simulink model "simulation"  (R2016a)
settings: Solver=VariableStepAuto  StartTime=0.0  StopTime=0.4  MaxStep=0.01  RelTol=1e-4
settings Model: Creator=michael  LastModifiedBy=michael
settings DataIOCC: LimitDataPoints=on  SaveOutput=off  SaveTime=off
settings OptimizationCC: ExpressionDepthLimit=2147483647  LifeSpan=1
settings DebuggingCC: UnderspecifiedInitializationDetection=Classic  MergeDetectMultiDrivingBlocksExec=none  FcnCallInpInsideContextMsg=EnableAllAsWarning  AllowSymbolicDim=off  StateNameClashWarn=warning
settings GRTTargetCC: CombineOutputUpdateFcns=off  GRTInterface=on

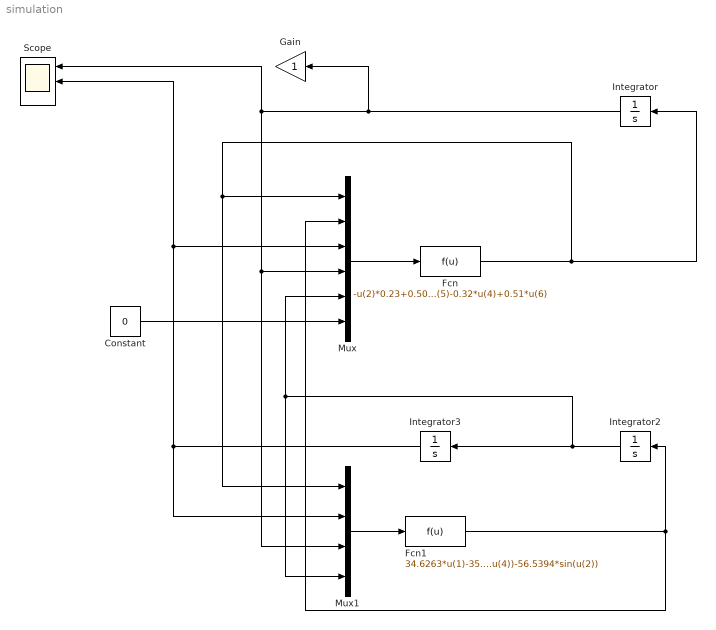
== system simulation ==
  Constant : Constant  Value=0
  Fcn : Fcn  Expr=-u(2)*0.23+0.505*(2*cos(u(3))-u(5)*sin(2*u(3))/cos(u(3)))+0.92*u(5)-0.32*u(4)+0.51*u(6)
  Fcn1 : Fcn  Expr=34.6263*u(1)-35.1227*cos(u(2))*u(1)-12.03945*(u(3)+u(4))-56.5394*sin(u(2))
  Gain : Gain
  Integrator : Integrator  InitialCondition=8.11
  Integrator2 : Integrator
  Integrator3 : Integrator
  Mux : Mux  Inputs=6
  Mux1 : Mux
  Scope : Scope  NumInputPorts=3
  wires:
  Mux1/1 -> Fcn1/1
  Mux/1 -> Fcn/1
  Fcn/1 -> Mux1/1, Mux/1, Integrator/1
  Fcn1/1 -> Integrator2/1, Mux/2
  Integrator2/1 -> Integrator3/1, Mux/5, Mux1/4
  Integrator/1 -> Gain/1, Mux1/3, Mux/4, Scope/1
  Constant/1 -> Mux/6
  Integrator3/1 -> Mux1/2, Scope/2, Mux/3
